simulink model "PEMFC_smlkCH4"  (R2015b)
settings: Solver=VariableStepAuto  StartTime=0.0  StopTime=tf  MinStep=1e-6  RelTol=1e-3
values from neighbouring files (symbols this model uses):
  A_cell = 238    [PEMFC_H2O2polarization.m]    (also in PEMFC_begin.m)
  B = 0.016    [PEMFC_CH4data.m]    (also in PEMFC_H2O2data.m = 0.005; PEMFC_H2O2polarization.m = 0.005; PEMFC_H2O2polfitting.m = 0.005; PEMFC_H2data.m)
  c_cw = 4.18e03    (= 4180)    [PEMFC_CH4data.m]    (also in PEMFC_H2O2data.m; PEMFC_H2data.m)
  c_O2 = p_O2 / (5.08e06 * exp(-498 / T))    [PEMFC_CH4data.m]    (also in PEMFC_H2O2data.m = pO2avg / (5.08e06 * exp(-498 / T)); PEMFC_H2O2polarization.m = pO2avg / (5.08e06 * exp(-498 / T(i))); PEMFC_H2O2polfitting.m = pO2avg / (5.08e06 * exp(-498 / T(i))); PEMFC_H2data.m)
  C_th = 350e03    (= 350000)    [PEMFC_CH4data.m]    (also in PEMFC_H2O2data.m; PEMFC_H2data.m)
  chi1 = 0.00129697    [PEMFC_CH4data.m]    (also in PEMFC_H2O2data.m; PEMFC_H2data.m)
  chi2 = - 1.529053    (= -1.529053)    [PEMFC_CH4data.m]    (also in PEMFC_H2O2data.m; PEMFC_H2data.m)
  chi3 = 681.731481    [PEMFC_CH4data.m]    (also in PEMFC_H2O2data.m; PEMFC_H2data.m)
  chi4 = - 136025.0    (= -136025)    [PEMFC_CH4data.m]    (also in PEMFC_H2O2data.m; PEMFC_H2data.m)
  chi5 = 10234070.7    [PEMFC_CH4data.m]    (also in PEMFC_H2O2data.m; PEMFC_H2data.m)
  CV = 4 * eta_ref    (= 3.92)    [PEMFC_CH4data.m]
  eta_ACDC = 0.92    [PEMFC_CH4data.m]    (also in PEMFC_H2data.m)
  eta_hx = 0.97    [PEMFC_CH4data.m]    (also in PEMFC_H2data.m = 0.92)
  F = 96485    [PEMFC_H2O2polarization.m]    (also in PEMFC_begin.m; PEMFC_cellstack.m)
  F_H2O = 0.5    [PEMFC_CH4data.m]    (also in PEMFC_H2data.m)
  h_airc = gamma_air * R * T / (gamma_air - 1) * ((1 / beta_c)^     ((gamma_air - 1) / gamma_air) - 1) / eta_c    [PEMFC_CH4data.m]    (also in PEMFC_H2data.m)
  h_airph = C_air * (T - T_amb) * M_air / eta_ph    [PEMFC_CH4data.m]    (also in PEMFC_H2data.m)
  h_CH4c = gamma_CH4 * R * T / (gamma_CH4 - 1) * ((1 / beta_c)^     ((gamma_CH4 - 1) / gamma_CH4) - 1) / eta_c    [PEMFC_CH4data.m]
  h_CH4ref = (h_CH4out - h_CH4in) / 0.97 * M_CH4    [PEMFC_CH4data.m]
  h_CO2pc = (h_CO2comb - h_CO2exh) / 1000 * M_CO2    [PEMFC_CH4data.m]
  h_CO2rec = (h_CO2rec_in - h_CO2_T) / 1000 * M_CO2 * eta_ref    [PEMFC_CH4data.m]
  h_cond = 500    [PEMFC_CH4data.m]    (also in PEMFC_H2O2data.m; PEMFC_H2data.m)
  h_conv = 0.1    [PEMFC_CH4data.m]    (also in PEMFC_H2O2data.m; PEMFC_H2data.m)
  h_H2Opc = C_H2Ocomb * (Tcomb - Texh) / 1000 * M_H2O    [PEMFC_CH4data.m]    (also in PEMFC_H2data.m)
  h_H2Opcvap = WaterEnthalpyVaporization (pcomb, T)    [PEMFC_CH4data.m]    (also in PEMFC_H2data.m)
  h_H2Orec = C_H2Orec * (T_ref - T) / 1000 * M_CO2 * eta_ref    [PEMFC_CH4data.m]
  h_H2Oref = (h_H2Oref_out - h_H2Oref_in) / 0.97 * M_H2O    [PEMFC_CH4data.m]
  h_H2rec = (h_H2rec_in - h_H2_T) / 1000 * M_CO2 * eta_ref    [PEMFC_CH4data.m]
  h_N2pc = (h_N2comb - h_N2exh) / 1000 * M_H2    [PEMFC_CH4data.m]    (also in PEMFC_H2data.m)
  h_O2pc = (h_O2comb - h_O2exh) / 1000 * M_O2    [PEMFC_CH4data.m]    (also in PEMFC_H2data.m)
  h_ref = - h_CH4ref - h_COref    (= 165000)    [PEMFC_CH4data.m]
  h_WHSG = h_H2OWH + h_H2Ovap    [PEMFC_CH4data.m]    (also in PEMFC_H2data.m)
  i_max = 1.2    [PEMFC_CH4data.m]    (also in PEMFC_H2O2data.m = 2.027; PEMFC_H2data.m; PEMFC_cellstack.m = 1.5)
  K_H2 = 0.04220    (= 0.0422)    [PEMFC_CH4data.m]    (also in PEMFC_H2O2data.m = pH2out / nH2out; PEMFC_H2data.m)
  K_O2 = 0.02110    (= 0.0211)    [PEMFC_CH4data.m]    (also in PEMFC_H2O2data.m = pO2out / nO2out; PEMFC_H2data.m)
  K_r = N_cell / (4 * F)    [PEMFC_CH4data.m]    (also in PEMFC_H2O2data.m; PEMFC_H2data.m)
  lambda = 0.90    (= 0.9)    [PEMFC_begin.m]
  m_cw = 0.25000    (= 0.25)    [PEMFC_CH4data.m]    (also in PEMFC_H2O2data.m; PEMFC_H2data.m)
  M_H2O = 18    [PEMFC_CH4data.m]    (also in PEMFC_H2O2data.m; PEMFC_H2data.m)
  N_cell = 178    [PEMFC_H2O2polarization.m]    (also in PEMFC_begin.m)
  p_cat = p_atm * 3.50    (= 3.5)    [PEMFC_H2O2polarization.m]    (also in PEMFC_begin.m)
  P_gamma = 150.0    (= 150)    [PEMFC_CH4data.m]    (also in PEMFC_H2O2data.m = 100; PEMFC_H2data.m = 155)
  p_H20 = y_H2_ref * p_an    [PEMFC_CH4data.m]    (also in PEMFC_H2O2data.m = (1 - xH2O_H2) * p_an; PEMFC_H2O2polarization.m = (1 - xH2O_H2) * p_an; PEMFC_H2O2polfitting.m = (1 - xH2O_H2) * p_an; PEMFC_H2data.m)
  p_O20 = x_O2 * p_cat    [PEMFC_CH4data.m]    (also in PEMFC_H2O2data.m = (1 - xH2O_O2) * p_cat; PEMFC_H2O2polarization.m = (1 - xH2O_O2) * p_cat; PEMFC_H2O2polfitting.m = (1 - xH2O_O2) * p_cat; PEMFC_H2data.m)
  psi = 23    [PEMFC_CH4data.m]    (also in PEMFC_H2O2data.m; PEMFC_H2O2polarization.m; PEMFC_H2O2polfitting.m; PEMFC_H2data.m)
  R_el = 0.00016    [PEMFC_CH4data.m]    (also in PEMFC_H2O2data.m = 0.00025492; PEMFC_H2data.m)
  R_th = 0.0817    [PEMFC_CH4data.m]    (also in PEMFC_H2O2data.m; PEMFC_H2data.m)
  SC = 2.50    (= 2.5)    [PEMFC_CH4data.m]
  split_CH4 = 0.30    (= 0.3)    [PEMFC_CH4data.m]
  T = [25 35 55 75 95] + 273.15    [PEMFC_H2O2polarization.m]    (also in PEMFC_begin.m = 347.15)
  T0 = T_a    [PEMFC_CH4data.m]    (also in PEMFC_H2O2data.m; PEMFC_H2data.m)
  T_a = 25    [PEMFC_begin.m]
  T_cwin = 20 + 0    (= 20)    [PEMFC_CH4data.m]    (also in PEMFC_H2O2data.m; PEMFC_H2data.m)
  T_des = T - 273.15    [PEMFC_CH4data.m]    (also in PEMFC_H2O2data.m; PEMFC_H2data.m)
  tau1_ref = 2.00    (= 2)    [PEMFC_CH4data.m]
  tau2_ref = 2.00    (= 2)    [PEMFC_CH4data.m]
  tau_c = 0.10    (= 0.1)    [PEMFC_CH4data.m]    (also in PEMFC_H2data.m)
  tau_H2 = 3.37    [PEMFC_CH4data.m]    (also in PEMFC_H2O2data.m = 0.27; PEMFC_H2data.m)
  tau_hx = 15.0    (= 15)    [PEMFC_CH4data.m]    (also in PEMFC_H2data.m)
  tau_O2 = 6.74    [PEMFC_CH4data.m]    (also in PEMFC_H2O2data.m = 0.47; PEMFC_H2data.m)
  tau_ph = 2.00    (= 2)    [PEMFC_CH4data.m]    (also in PEMFC_H2data.m = 3)
  tau_th = C_th * R_th    (= 28595)    [PEMFC_CH4data.m]    (also in PEMFC_H2O2data.m; PEMFC_H2data.m)
  tau_WHSG = 40.00    (= 40)    [PEMFC_CH4data.m]    (also in PEMFC_H2data.m = 50)
  U = polyval(polU, n_CH4in(1))    [PEMFC_CH4data.m]    (also in PEMFC_H2O2polarization.m = extractfield(V, b2)'; PEMFC_H2O2polfitting.m = extractfield(V, b2)'; PEMFC_H2data.m = polyval(polU, n_H2in(1)))
  V_tn = 1.48    [PEMFC_CH4data.m]    (also in PEMFC_H2O2data.m = 1.253; PEMFC_H2data.m)
  x_H2O = p_H2Ovap / p_cat    [PEMFC_CH4data.m]    (also in PEMFC_H2data.m)
  x_H2Ovap = WaterSaturationPressure (Texh) / pcomb    [PEMFC_CH4data.m]    (also in PEMFC_H2data.m)
  x_O2 = 0.21    [PEMFC_begin.m]
  xi1 = -0.949    [PEMFC_CH4data.m]    (also in PEMFC_H2O2data.m = -0.61693; PEMFC_H2O2polarization.m = xi(1); PEMFC_H2data.m; PEMFC_cellstack.m)
  xi2 = 0.003420    (= 0.00342)    [PEMFC_CH4data.m]    (also in PEMFC_H2O2data.m = 0.0016838; PEMFC_H2O2polarization.m = xi(2); PEMFC_H2data.m; PEMFC_cellstack.m)
  xi3 = 7.6e-05    [PEMFC_CH4data.m]    (also in PEMFC_H2O2data.m = 1.9385e-06; PEMFC_H2O2polarization.m = xi(3); PEMFC_H2data.m; PEMFC_cellstack.m)
  xi4 = -1.93e-04    (= -0.000193)    [PEMFC_CH4data.m]    (also in PEMFC_H2O2data.m = -6.4922e-05; PEMFC_H2O2polarization.m = xi(4); PEMFC_H2data.m; PEMFC_cellstack.m)
  y_CO2_ref = 1 - y_H2_ref - y_H2O_ref    [PEMFC_CH4data.m]    (also in PEMFC_H2data.m)
  y_H2_ref = 0.66    [PEMFC_begin.m]
  y_H2O_ref = 0.15    [PEMFC_begin.m]
  z_m = 178e-04    (= 0.0178)    [PEMFC_CH4data.m]    (also in PEMFC_H2O2polarization.m = 0.003; PEMFC_H2data.m; PEMFC_begin.m = 0.003; PEMFC_cellstack.m)
settings Model: Creator=gapaolo  LastModifiedBy=gapaolo

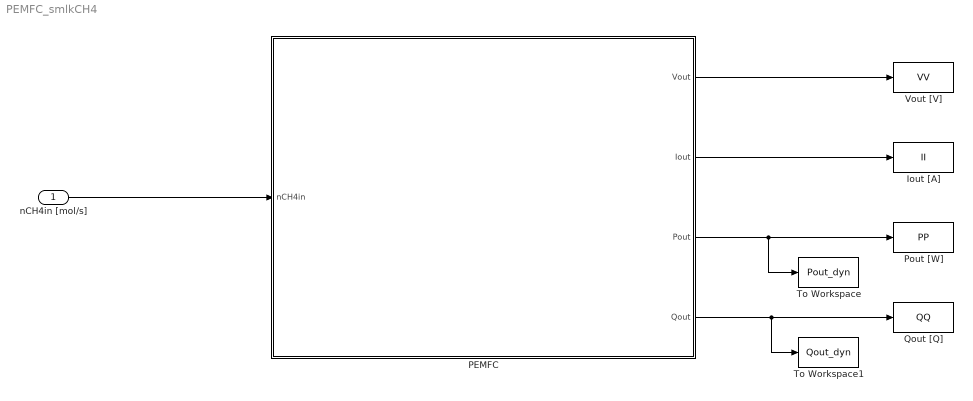
== system PEMFC_smlkCH4 ==
  nCH4in [mol/s] : Inport
  Iout [A] : ToWorkspace  VariableName=II  SaveFormat=Timeseries  SampleTime=-1
  PEMFC : Subsystem
  Pout [W] : ToWorkspace  VariableName=PP  SaveFormat=Timeseries  SampleTime=-1
  Qout [Q] : ToWorkspace  VariableName=QQ  SaveFormat=Timeseries  SampleTime=-1
  To Workspace : ToWorkspace  VariableName=Pout_dyn  SaveFormat=Timeseries  SampleTime=-1
  To Workspace1 : ToWorkspace  VariableName=Qout_dyn  SaveFormat=Timeseries  SampleTime=-1
  Vout [V] : ToWorkspace  VariableName=VV  SaveFormat=Timeseries  SampleTime=-1
  wires:
  nCH4in [mol/s]/1 -> PEMFC/1(nCH4in)
  PEMFC/1(Vout) -> Vout [V]/1
  PEMFC/2(Iout) -> Iout [A]/1
  PEMFC/4(Qout) -> To Workspace1/1, Qout [Q]/1
  PEMFC/3(Pout) -> To Workspace/1, Pout [W]/1

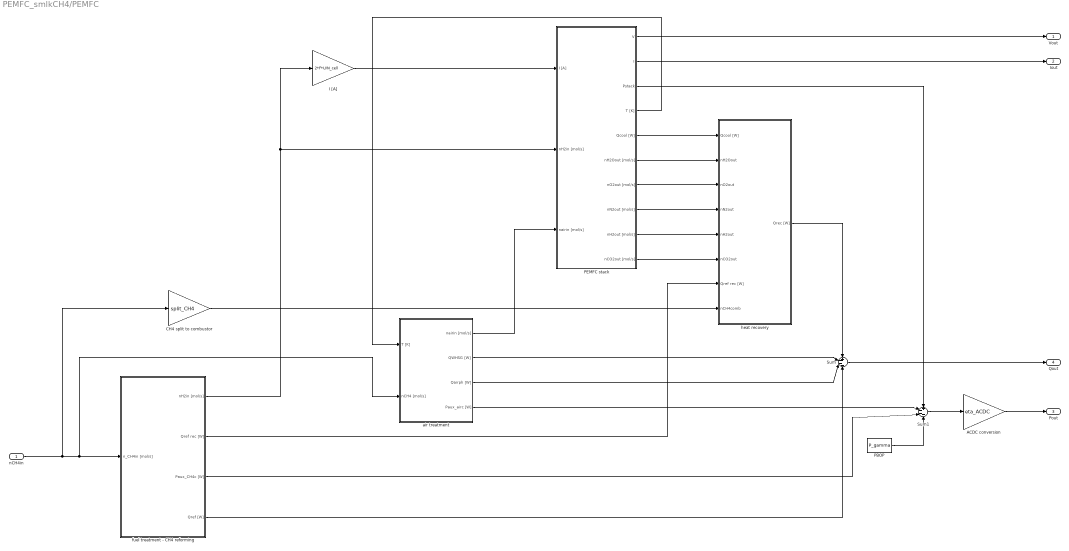
== system PEMFC_smlkCH4/PEMFC ==
  nCH4in : Inport
  ACDC conversion : Gain  Gain=eta_ACDC
  CH4 split to combustor : Gain  Gain=split_CH4
  I [A] : Gain  Gain=2*F*U/N_cell
  PBOP : Constant  Value=P_gamma
  PEMFC stack : Subsystem
  Sum : Sum  Inputs=+---
  Sum1 : Sum  Inputs=+---
  air treatment : Subsystem
  fuel treatment - CH4 reforming : Subsystem
  heat recovery : Subsystem
  Vout : Outport
  Iout : Outport  Port=2
  Pout : Outport  Port=3
  Qout : Outport  Port=4
  wires:
  fuel treatment - CH4 reforming/1(nH2in [mol/s]) -> I [A]/1, PEMFC stack/2(nH2in [mol/s])
  I [A]/1 -> PEMFC stack/1(I [A])
  air treatment/1(nairin [mol/s]) -> PEMFC stack/3(nairin [mol/s])
  PEMFC stack/1("V ") -> Vout/1
  PEMFC stack/2(I) -> Iout/1
  PEMFC stack/4(T [K]) -> air treatment/1(T [K])
  PEMFC stack/3(Pstack) -> Sum1/1
  PEMFC stack/5(Qcool [W]) -> heat recovery/1(Qcool [W])
  fuel treatment - CH4 reforming/2(Qref rec [W]) -> heat recovery/7(Qref rec [W])
  PEMFC stack/6(nH2Oout [mol/s]) -> heat recovery/2(nH2Oout)
  PEMFC stack/7(nO2out [mol/s]) -> heat recovery/3(nO2out)
  PEMFC stack/8(nN2out [mol/s]) -> heat recovery/4(nN2out)
  PEMFC stack/9(nH2out [mol/s]) -> heat recovery/5(nH2out)
  PEMFC stack/10(nCO2out [mol/s]) -> heat recovery/6(nCO2out)
  CH4 split to combustor/1 -> heat recovery/8(nCH4comb)
  Sum1/1 -> ACDC conversion/1
  heat recovery/1(Qrec [W]) -> Sum/1
  fuel treatment - CH4 reforming/3(Paux_CH4c [W]) -> Sum1/3
  air treatment/3(Qairph [W]) -> Sum/3
  air treatment/4(Paux_airc [W]) -> Sum1/2
  air treatment/2(QWHSG [W]) -> Sum/2
  fuel treatment - CH4 reforming/4(Qref [W]) -> Sum/4
  nCH4in/1 -> CH4 split to combustor/1, air treatment/2(nCH4 [mol/s]), fuel treatment - CH4 reforming/1(n_CH4in [mol/s])
  PBOP/1 -> Sum1/4
  ACDC conversion/1 -> Pout/1
  Sum/1 -> Qout/1

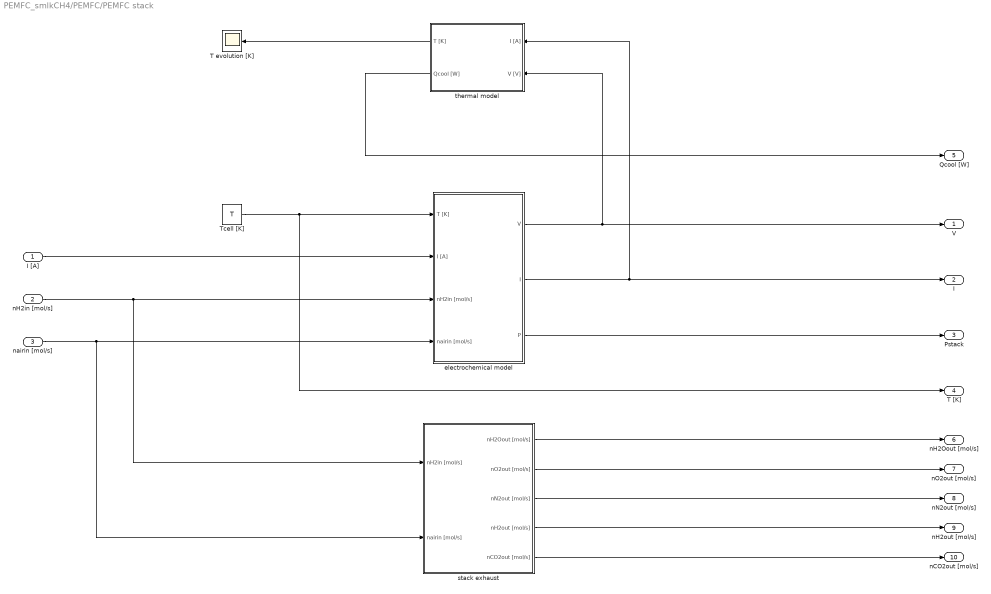
== system PEMFC_smlkCH4/PEMFC/PEMFC stack ==
  I [A] : Inport
  nH2in [mol/s] : Inport  Port=2
  nairin [mol/s] : Inport  Port=3
  T evolution [K] : Scope
  Tcell [K] : Constant  Value=T
  electrochemical model : Subsystem
  stack exhaust : Subsystem
  thermal model : Subsystem
  "V " : Outport
  I : Outport  Port=2
  Pstack : Outport  Port=3
  T [K] : Outport  Port=4
  Qcool [W] : Outport  Port=5
  nH2Oout [mol/s] : Outport  Port=6
  nO2out [mol/s] : Outport  Port=7
  nN2out [mol/s] : Outport  Port=8
  nH2out [mol/s] : Outport  Port=9
  nCO2out [mol/s] : Outport  Port=10
  wires:
  nairin [mol/s]/1 -> stack exhaust/2(nairin [mol/s]), electrochemical model/4(nairin [mol/s])
  electrochemical model/3(P) -> Pstack/1
  nH2in [mol/s]/1 -> electrochemical model/3(nH2in [mol/s]), stack exhaust/1(nH2in [mol/s])
  stack exhaust/1(nH2Oout [mol/s]) -> nH2Oout [mol/s]/1
  stack exhaust/2(nO2out [mol/s]) -> nO2out [mol/s]/1
  stack exhaust/3(nN2out [mol/s]) -> nN2out [mol/s]/1
  stack exhaust/4(nH2out [mol/s]) -> nH2out [mol/s]/1
  stack exhaust/5(nCO2out [mol/s]) -> nCO2out [mol/s]/1
  Tcell [K]/1 -> T [K]/1, electrochemical model/1(T [K])
  thermal model/1(T [K]) -> T evolution [K]/1
  I [A]/1 -> electrochemical model/2("I [A] ")
  thermal model/2(Qcool [W]) -> Qcool [W]/1
  electrochemical model/2(I) -> I/1, thermal model/1(I [A])
  electrochemical model/1(V) -> thermal model/2(V [V]), "V "/1

== system PEMFC_smlkCH4/PEMFC/air treatment ==
  T [K] : Inport
  nCH4 [mol/s] : Inport  Port=2
  CH4 --> H2 : Gain  Gain=CV
  Sum1 : Sum  Inputs=++|
  Water vaporization : Subsystem
  air humdifier : Subsystem
  auxiliaries - air compressor and preheater : Subsystem
  nairin [mol/s] : Outport
  QWHSG [W] : Outport  Port=2
  Qairph [W] : Outport  Port=3
  Paux_airc [W] : Outport  Port=4
  wires:
  nCH4 [mol/s]/1 -> CH4 --> H2/1
  T [K]/1 -> air humdifier/2(T [K])
  air humdifier/2(nair dry [mol/s]) -> auxiliaries - air compressor and preheater/1(nair dry [mol/s])
  auxiliaries - air compressor and preheater/2(Qairph [W]) -> Qairph [W]/1
  auxiliaries - air compressor and preheater/3(Paux_airc [W]) -> Paux_airc [W]/1
  auxiliaries - air compressor and preheater/1(nair dry) -> Sum1/2
  Sum1/1 -> nairin [mol/s]/1
  air humdifier/1(nH2O [mol/s]) -> Water vaporization/1(nH2O [mol/s])
  Water vaporization/1(QWHSG) -> QWHSG [W]/1
  Water vaporization/2(nH2O) -> Sum1/1
  CH4 --> H2/1 -> air humdifier/1(nH2 [mol/s])

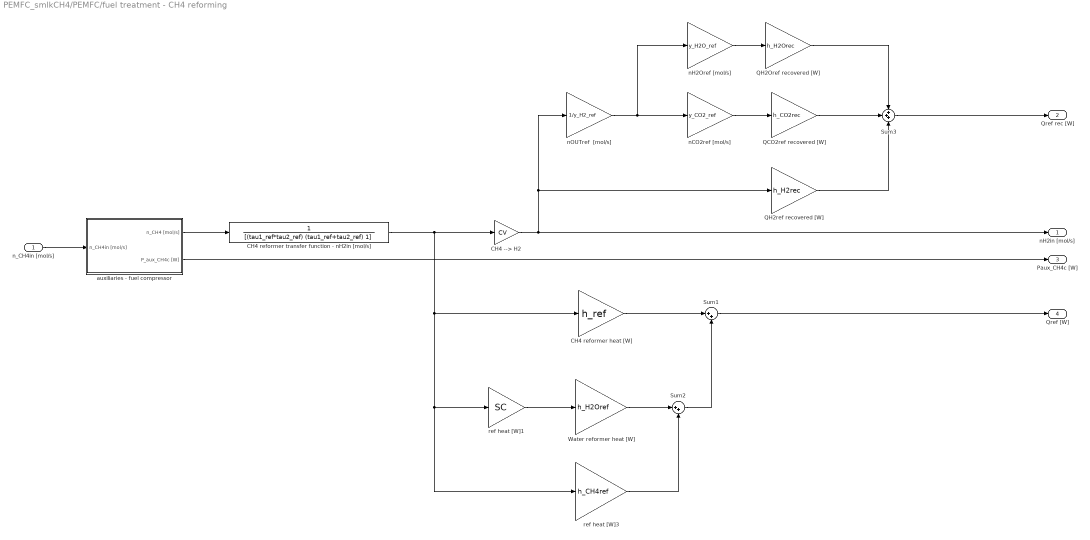
== system PEMFC_smlkCH4/PEMFC/fuel treatment - CH4 reforming ==
  n_CH4in [mol/s] : Inport
  CH4 --> H2 : Gain  Gain=CV
  CH4 reformer heat [W] : Gain  Gain=h_ref
  CH4 reformer transfer function - nH2in [mol/s] : TransferFcn  Denominator=[(tau1_ref*tau2_ref) (tau1_ref+tau2_ref) 1]  ContinuousStateAttributes='q_H2'
  QCO2ref recovered [W] : Gain  Gain=h_CO2rec
  QH2Oref recovered [W] : Gain  Gain=h_H2Orec
  QH2ref recovered [W] : Gain  Gain=h_H2rec
  Sum1 : Sum  Inputs=|++
  Sum2 : Sum  Inputs=|++
  Sum3 : Sum  Inputs=+++
  Water reformer heat [W] : Gain  Gain=h_H2Oref
  auxiliaries - fuel compressor : Subsystem
  nCO2ref [mol/s] : Gain  Gain=y_CO2_ref
  nH2Oref [mol/s] : Gain  Gain=y_H2O_ref
  "nOUTref  [mol/s] " : Gain  Gain=1/y_H2_ref
  ref heat [W]1 : Gain  Gain=SC
  ref heat [W]3 : Gain  Gain=h_CH4ref
  nH2in [mol/s] : Outport
  Qref rec [W] : Outport  Port=2
  Paux_CH4c [W] : Outport  Port=3
  Qref [W] : Outport  Port=4
  wires:
  CH4 reformer transfer function - nH2in [mol/s]/1 -> ref heat [W]3/1, ref heat [W]1/1, CH4 reformer heat [W]/1, CH4 --> H2/1
  auxiliaries - fuel compressor/2(P_aux_CH4c [W]) -> Paux_CH4c [W]/1
  CH4 --> H2/1 -> "nOUTref  [mol/s] "/1, QH2ref recovered [W]/1, nH2in [mol/s]/1
  auxiliaries - fuel compressor/1(n_CH4 [mol/s]) -> CH4 reformer transfer function - nH2in [mol/s]/1
  Sum2/1 -> Sum1/2
  ref heat [W]3/1 -> Sum2/2
  ref heat [W]1/1 -> Water reformer heat [W]/1
  CH4 reformer heat [W]/1 -> Sum1/1
  Water reformer heat [W]/1 -> Sum2/1
  Sum1/1 -> Qref [W]/1
  n_CH4in [mol/s]/1 -> auxiliaries - fuel compressor/1(n_CH4in [mol/s])
  "nOUTref  [mol/s] "/1 -> nH2Oref [mol/s]/1, nCO2ref [mol/s]/1
  nH2Oref [mol/s]/1 -> QH2Oref recovered [W]/1
  nCO2ref [mol/s]/1 -> QCO2ref recovered [W]/1
  QCO2ref recovered [W]/1 -> Sum3/2
  QH2Oref recovered [W]/1 -> Sum3/1
  QH2ref recovered [W]/1 -> Sum3/3
  Sum3/1 -> Qref rec [W]/1

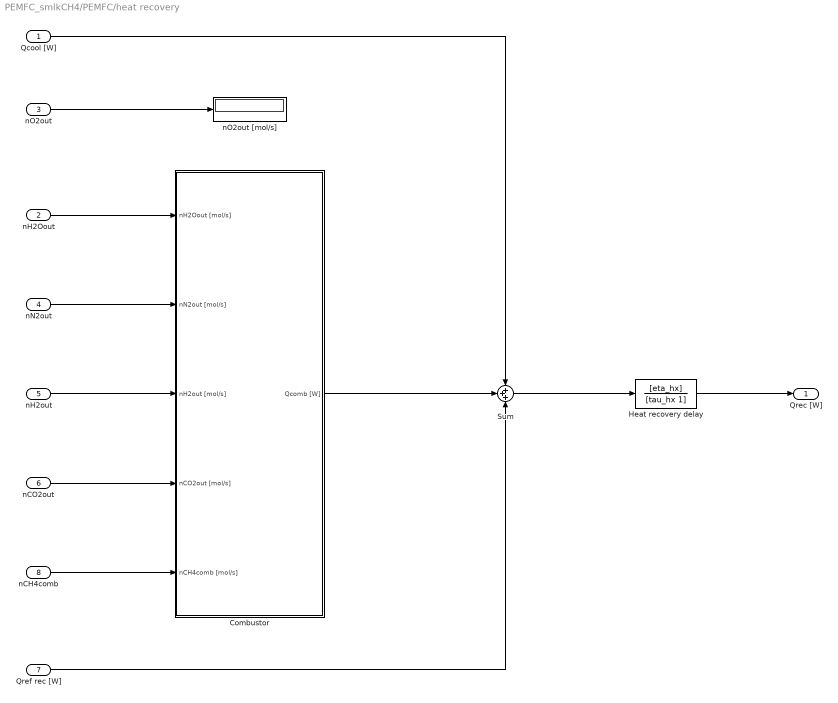
== system PEMFC_smlkCH4/PEMFC/heat recovery ==
  Qcool [W] : Inport
  nH2Oout : Inport  Port=2
  nO2out : Inport  Port=3
  nN2out : Inport  Port=4
  nH2out : Inport  Port=5
  nCO2out : Inport  Port=6
  Qref rec [W] : Inport  Port=7
  nCH4comb : Inport  Port=8
  Combustor : Subsystem
  Heat recovery delay : TransferFcn  Numerator=[eta_hx]  Denominator=[tau_hx 1]
  Sum : Sum  Inputs=+++
  nO2out [mol/s] : Display
  Qrec [W] : Outport
  wires:
  nO2out/1 -> nO2out [mol/s]/1
  nH2Oout/1 -> Combustor/1(nH2Oout [mol/s])
  nN2out/1 -> Combustor/2(nN2out [mol/s])
  nH2out/1 -> Combustor/3(nH2out [mol/s])
  nCO2out/1 -> Combustor/4(nCO2out [mol/s])
  nCH4comb/1 -> Combustor/5(nCH4comb [mol/s])
  Combustor/1(Qcomb [W]) -> Sum/2
  Qref rec [W]/1 -> Sum/3
  Qcool [W]/1 -> Sum/1
  Sum/1 -> Heat recovery delay/1
  Heat recovery delay/1 -> Qrec [W]/1

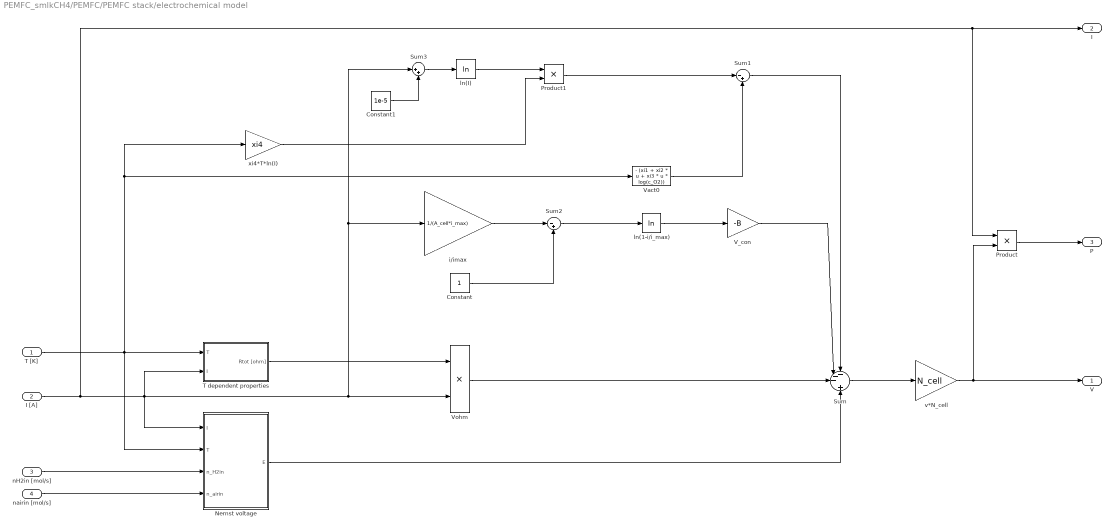
== system PEMFC_smlkCH4/PEMFC/PEMFC stack/electrochemical model ==
  T [K] : Inport
  "I [A] " : Inport  Port=2
  nH2in [mol/s] : Inport  Port=3
  nairin [mol/s] : Inport  Port=4
  Constant : Constant
  Constant1 : Constant  Value=1e-5
  Nernst voltage : Subsystem
  Product : Product
  Product1 : Product
  Sum : Sum  Inputs=---|+
  Sum1 : Sum  Inputs=|-+
  Sum2 : Sum  Inputs=|-+
  Sum3 : Sum  Inputs=|++
  T dependent properties : Subsystem
  V_con : Gain  Gain=-B
  Vact0 : Fcn  Expr=- (xi1 + xi2 * u + xi3 * u * log(c_O2))
  Vohm : Product
  i/imax : Gain  Gain=1/(A_cell*i_max)
  ln(1-i/i_max) : Math  Operator=log  SaturateOnIntegerOverflow=on
  "ln(I) " : Math  Operator=log  SaturateOnIntegerOverflow=on
  v*N_cell : Gain  Gain=N_cell
  xi4*T*ln(I) : Gain  Gain=xi4
  V : Outport
  I : Outport  Port=2
  P : Outport  Port=3
  wires:
  Sum/1 -> v*N_cell/1
  T [K]/1 -> xi4*T*ln(I)/1, Vact0/1, Nernst voltage/2(T), T dependent properties/1(T)
  T dependent properties/1(Rtot [ohm]) -> Vohm/1
  Vohm/1 -> Sum/3
  i/imax/1 -> Sum2/1
  Constant/1 -> Sum2/2
  Sum2/1 -> ln(1-i/i_max)/1
  ln(1-i/i_max)/1 -> V_con/1
  Sum1/1 -> Sum/1
  v*N_cell/1 -> Product/2, V/1
  V_con/1 -> Sum/2
  "ln(I) "/1 -> Product1/1
  Product1/1 -> Sum1/1
  Vact0/1 -> Sum1/2
  "I [A] "/1 -> Product/1, I/1, Nernst voltage/1(I), T dependent properties/2(I), Vohm/2, i/imax/1, Sum3/1
  Nernst voltage/1(E) -> Sum/4
  nH2in [mol/s]/1 -> Nernst voltage/3(n_H2in)
  nairin [mol/s]/1 -> Nernst voltage/4(n_airin)
  Product/1 -> P/1
  Sum3/1 -> "ln(I) "/1
  Constant1/1 -> Sum3/2
  xi4*T*ln(I)/1 -> Product1/2

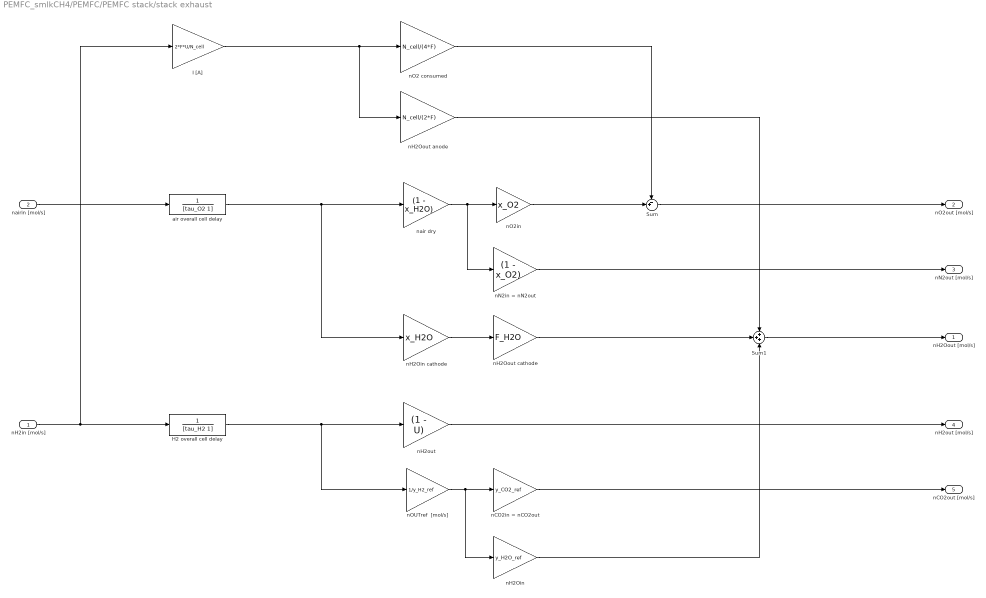
== system PEMFC_smlkCH4/PEMFC/PEMFC stack/stack exhaust ==
  nH2in [mol/s] : Inport
  nairin [mol/s] : Inport  Port=2
  H2 overall cell delay : TransferFcn  Denominator=[tau_H2 1]  ContinuousStateAttributes='p_O2'
  I [A] : Gain  Gain=2*F*U/N_cell
  Sum : Sum  Inputs=-+|
  Sum1 : Sum  Inputs=+++
  air overall cell delay : TransferFcn  Denominator=[tau_O2 1]  ContinuousStateAttributes='p_O2'
  nCO2in = nCO2out : Gain  Gain=y_CO2_ref
  nH2Oin : Gain  Gain=y_H2O_ref
  nH2Oin cathode : Gain  Gain=x_H2O
  nH2Oout anode : Gain  Gain=N_cell/(2*F)
  nH2Oout cathode : Gain  Gain=F_H2O
  nH2out : Gain  Gain=(1 - U)
  nN2in = nN2out : Gain  Gain=(1 - x_O2)
  nO2 consumed : Gain  Gain=N_cell/(4*F)
  nO2in : Gain  Gain=x_O2
  "nOUTref  [mol/s] " : Gain  Gain=1/y_H2_ref
  nair dry : Gain  Gain=(1 - x_H2O)
  nH2Oout [mol/s] : Outport
  nO2out [mol/s] : Outport  Port=2
  nN2out [mol/s] : Outport  Port=3
  nH2out [mol/s] : Outport  Port=4
  nCO2out [mol/s] : Outport  Port=5
  wires:
  nH2Oin cathode/1 -> nH2Oout cathode/1
  nair dry/1 -> nN2in = nN2out/1, nO2in/1
  nairin [mol/s]/1 -> air overall cell delay/1
  nH2in [mol/s]/1 -> I [A]/1, H2 overall cell delay/1
  nO2in/1 -> Sum/2
  nO2 consumed/1 -> Sum/1
  "nOUTref  [mol/s] "/1 -> nH2Oin/1, nCO2in = nCO2out/1
  Sum/1 -> nO2out [mol/s]/1
  nH2Oout cathode/1 -> Sum1/2
  nH2Oout anode/1 -> Sum1/1
  nH2Oin/1 -> Sum1/3
  Sum1/1 -> nH2Oout [mol/s]/1
  nN2in = nN2out/1 -> nN2out [mol/s]/1
  nH2out/1 -> nH2out [mol/s]/1
  nCO2in = nCO2out/1 -> nCO2out [mol/s]/1
  H2 overall cell delay/1 -> "nOUTref  [mol/s] "/1, nH2out/1
  air overall cell delay/1 -> nH2Oin cathode/1, nair dry/1
  I [A]/1 -> nH2Oout anode/1, nO2 consumed/1

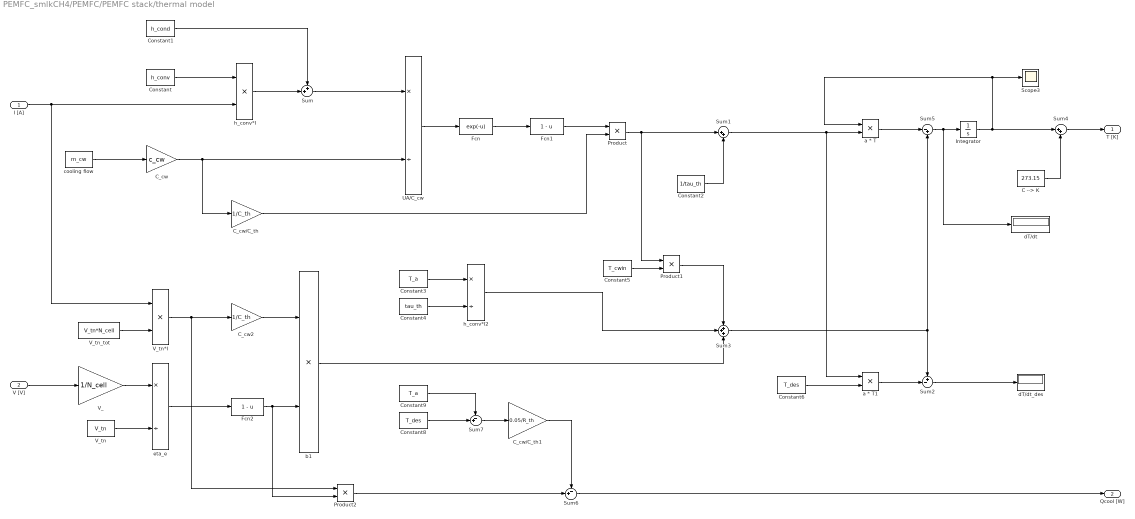
== system PEMFC_smlkCH4/PEMFC/PEMFC stack/thermal model ==
  I [A] : Inport
  V [V] : Inport  Port=2
  C --> K : Constant  Value=273.15
  C_cw : Gain  Gain=c_cw
  C_cw/C_th : Gain  Gain=1/C_th
  C_cw/C_th1 : Gain  Gain=0.05/R_th
  C_cw2 : Gain  Gain=1/C_th
  Constant : Constant  Value=h_conv
  Constant1 : Constant  Value=h_cond
  Constant2 : Constant  Value=1/tau_th
  Constant3 : Constant  Value=T_a
  Constant4 : Constant  Value=tau_th
  Constant5 : Constant  Value=T_cwin
  Constant6 : Constant  Value=T_des
  Constant8 : Constant  Value=T_des
  Constant9 : Constant  Value=T_a
  Fcn : Fcn  Expr=exp(-u)
  Fcn1 : Fcn  Expr=1 - u
  Fcn2 : Fcn  Expr=1 - u
  Integrator : Integrator  InitialCondition=T0  AbsoluteTolerance=1e-6
  Product : Product
  Product1 : Product
  Product2 : Product
  Scope3 : Scope
  Sum : Sum  Inputs=++|
  Sum1 : Sum  Inputs=|++
  Sum2 : Sum  Inputs=+-|
  Sum3 : Sum  Inputs=+++
  Sum4 : Sum  Inputs=|++
  Sum5 : Sum  Inputs=|-+
  Sum6 : Sum  Inputs=-+|
  Sum7 : Sum  Inputs=-+|
  UA/C_cw : Product  Inputs=*/
  V_ : Gain  Gain=1/N_cell
  V_tn : Constant  Value=V_tn
  V_tn*I : Product
  V_tn_tot : Constant  Value=V_tn*N_cell
  a * T : Product
  a * T1 : Product
  b1 : Product
  cooling flow : Constant  Value=m_cw
  dT/dt : Display
  dT/dt_des : Display
  eta_e : Product  Inputs=*/
  h_conv*I : Product
  h_conv*I2 : Product  Inputs=*/
  T [K] : Outport
  Qcool [W] : Outport  Port=2
  wires:
  V_tn_tot/1 -> V_tn*I/2
  eta_e/1 -> Fcn2/1
  V_tn/1 -> eta_e/2
  V_/1 -> eta_e/1
  b1/1 -> Sum3/3
  h_conv*I2/1 -> Sum3/2
  Product1/1 -> Sum3/1
  Constant5/1 -> Product1/2
  Constant4/1 -> h_conv*I2/2
  Constant3/1 -> h_conv*I2/1
  C_cw2/1 -> b1/1
  V [V]/1 -> V_/1
  Constant2/1 -> Sum1/2
  Product/1 -> Sum1/1, Product1/1
  C_cw/C_th/1 -> Product/2
  Fcn1/1 -> Product/1
  C_cw/1 -> C_cw/C_th/1, UA/C_cw/2
  Fcn/1 -> Fcn1/1
  UA/C_cw/1 -> Fcn/1
  cooling flow/1 -> C_cw/1
  Sum/1 -> UA/C_cw/1
  Constant1/1 -> Sum/1
  h_conv*I/1 -> Sum/2
  Constant/1 -> h_conv*I/1
  I [A]/1 -> h_conv*I/2, V_tn*I/1
  Integrator/1 -> Sum4/1, a * T/1, Scope3/1
  a * T/1 -> Sum5/1
  Sum3/1 -> Sum5/2, Sum2/1
  Sum1/1 -> a * T1/1, a * T/2
  Constant6/1 -> a * T1/2
  a * T1/1 -> Sum2/2
  Sum2/1 -> dT/dt_des/1
  C --> K/1 -> Sum4/2
  Sum4/1 -> T [K]/1
  Product2/1 -> Sum6/2
  Constant8/1 -> Sum7/2
  Constant9/1 -> Sum7/1
  Sum7/1 -> C_cw/C_th1/1
  C_cw/C_th1/1 -> Sum6/1
  Sum6/1 -> Qcool [W]/1
  V_tn*I/1 -> Product2/1, C_cw2/1
  Fcn2/1 -> Product2/2, b1/2
  Sum5/1 -> dT/dt/1, Integrator/1

== system PEMFC_smlkCH4/PEMFC/air treatment/Water vaporization ==
  nH2O [mol/s] : Inport
  Q_WHSG [W] : Gain  Gain=h_WHSG
  WHSG delay : TransferFcn  Denominator=[tau_WHSG 1]
  mH2O [g/s] : Gain  Gain=M_H2O
  nH2Odelay [mol/s] : Gain  Gain=1/h_WHSG/M_H2O
  QWHSG : Outport
  nH2O : Outport  Port=2
  wires:
  mH2O [g/s]/1 -> Q_WHSG [W]/1
  Q_WHSG [W]/1 -> WHSG delay/1
  nH2O [mol/s]/1 -> mH2O [g/s]/1
  WHSG delay/1 -> QWHSG/1, nH2Odelay [mol/s]/1
  nH2Odelay [mol/s]/1 -> nH2O/1

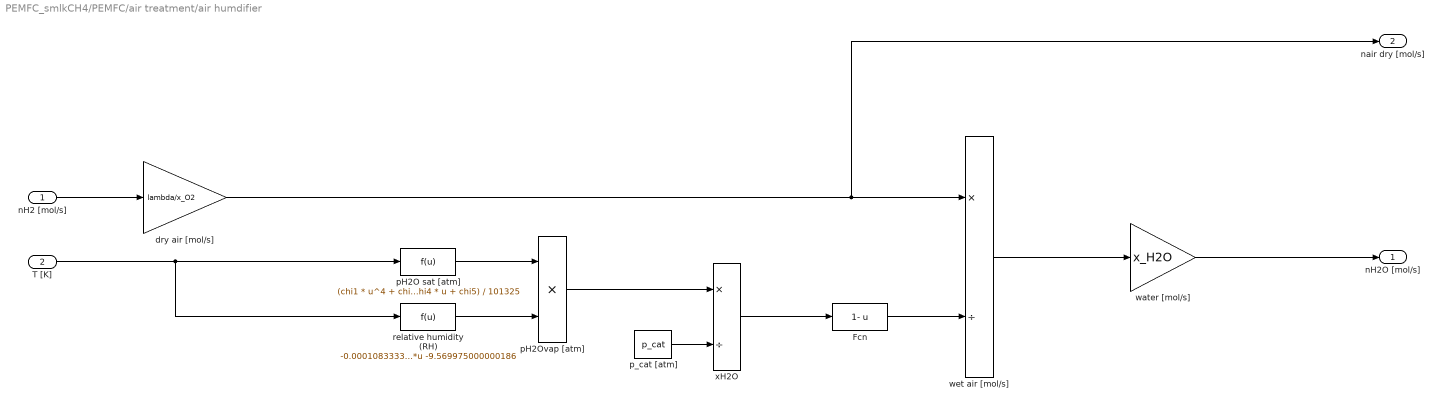
== system PEMFC_smlkCH4/PEMFC/air treatment/air humdifier ==
  nH2 [mol/s] : Inport
  T [K] : Inport  Port=2
  Fcn : Fcn  Expr=1- u
  dry air [mol/s] : Gain  Gain=lambda/x_O2
  pH2O sat [atm] : Fcn  Expr=(chi1 * u^4 + chi2 * u^3 + chi3 * u^2 + chi4 * u + chi5) / 101325
  pH2Ovap [atm] : Product
  p_cat [atm] : Constant  Value=p_cat
  relative humidity (RH) : Fcn  Expr=-0.000108333333333*u^2 + 0.067816666666668*u -9.569975000000186
  water [mol/s] : Gain  Gain=x_H2O
  wet air [mol/s] : Product  Inputs=*/
  xH2O : Product  Inputs=*/
  nH2O [mol/s] : Outport
  nair dry [mol/s] : Outport  Port=2
  wires:
  Fcn/1 -> wet air [mol/s]/2
  xH2O/1 -> Fcn/1
  dry air [mol/s]/1 -> nair dry [mol/s]/1, wet air [mol/s]/1
  wet air [mol/s]/1 -> water [mol/s]/1
  nH2 [mol/s]/1 -> dry air [mol/s]/1
  pH2Ovap [atm]/1 -> xH2O/1
  pH2O sat [atm]/1 -> pH2Ovap [atm]/1
  relative humidity (RH)/1 -> pH2Ovap [atm]/2
  p_cat [atm]/1 -> xH2O/2
  T [K]/1 -> relative humidity (RH)/1, pH2O sat [atm]/1
  water [mol/s]/1 -> nH2O [mol/s]/1

== system PEMFC_smlkCH4/PEMFC/air treatment/auxiliaries - air compressor and preheater ==
  nair dry [mol/s] : Inport
  Paux_airc : Gain  Gain=h_airc
  Qairph : Gain  Gain=h_airph
  air preheating delay : TransferFcn  Denominator=[tau_ph 1]
  nair dry delay : Gain  Gain=1/h_airph
  nair dry : Outport
  Qairph [W] : Outport  Port=2
  Paux_airc [W] : Outport  Port=3
  wires:
  nair dry [mol/s]/1 -> Qairph/1, Paux_airc/1
  Paux_airc/1 -> Paux_airc [W]/1
  Qairph/1 -> air preheating delay/1
  nair dry delay/1 -> nair dry/1
  air preheating delay/1 -> Qairph [W]/1, nair dry delay/1

== system PEMFC_smlkCH4/PEMFC/fuel treatment - CH4 reforming/auxiliaries - fuel compressor ==
  n_CH4in [mol/s] : Inport
  CH4 compression delay : TransferFcn  Denominator=[tau_c 1]
  CH4 compression work : Gain  Gain=h_CH4c
  CH4 mole flow : Gain  Gain=1/h_CH4c
  n_CH4 [mol/s] : Outport
  P_aux_CH4c [W] : Outport  Port=2
  wires:
  CH4 compression work/1 -> CH4 compression delay/1
  n_CH4in [mol/s]/1 -> CH4 compression work/1
  CH4 mole flow/1 -> n_CH4 [mol/s]/1
  CH4 compression delay/1 -> CH4 mole flow/1, P_aux_CH4c [W]/1

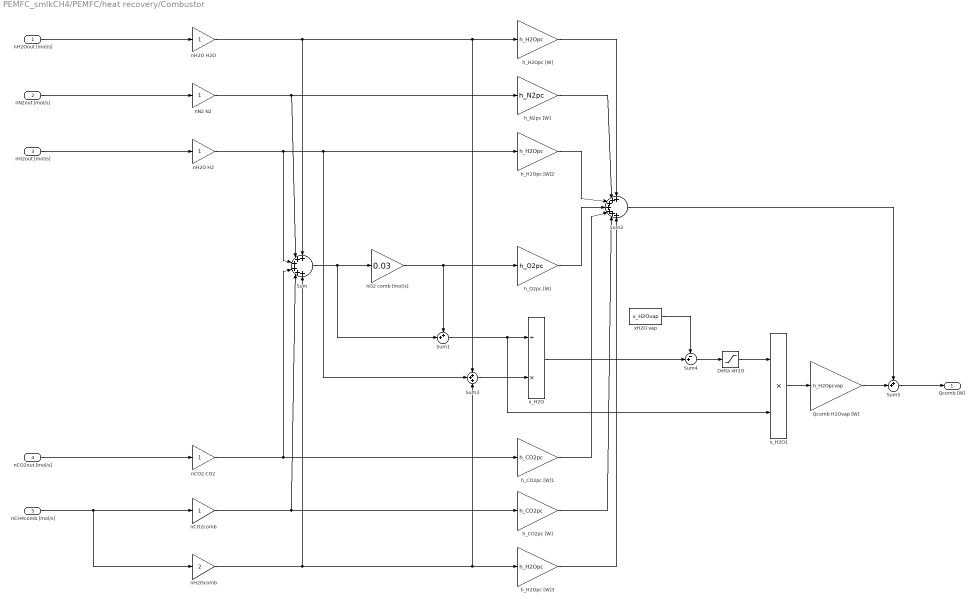
== system PEMFC_smlkCH4/PEMFC/heat recovery/Combustor ==
  nH2Oout [mol/s] : Inport
  nN2out [mol/s] : Inport  Port=2
  nH2out [mol/s] : Inport  Port=3
  nCO2out [mol/s] : Inport  Port=4
  nCH4comb [mol/s] : Inport  Port=5
  Delta xH2O : Saturate  UpperLimit=1  LowerLimit=0
  Qcomb H2Ovap [W] : Gain  Gain=h_H2Opcvap
  Sum : Sum  Inputs=++++++
  Sum1 : Sum  Inputs=++|
  Sum2 : Sum  Inputs=+++++++
  Sum3 : Sum  Inputs=+++
  Sum4 : Sum  Inputs=-+|
  Sum5 : Sum  Inputs=++|
  h_CO2pc [W] : Gain  Gain=h_CO2pc
  h_CO2pc [W]1 : Gain  Gain=h_CO2pc
  h_H2Opc [W] : Gain  Gain=h_H2Opc
  h_H2Opc [W]2 : Gain  Gain=h_H2Opc
  h_H2Opc [W]3 : Gain  Gain=h_H2Opc
  h_N2pc [W] : Gain  Gain=h_N2pc
  h_O2pc [W] : Gain  Gain=h_O2pc
  nCO2 CO2 : Gain
  nCO2comb : Gain
  nH2O H2 : Gain
  nH2O H2O : Gain
  nH2Ocomb : Gain  Gain=2
  nN2 N2 : Gain
  nO2 comb [mol/s] : Gain  Gain=0.03
  xH2O vap : Constant  Value=x_H2Ovap
  x_H2O : Product  Inputs=/*
  x_H2O1 : Product  Inputs=**
  Qcomb [W] : Outport
  wires:
  h_H2Opc [W]/1 -> Sum2/1
  Sum2/1 -> Sum5/1
  h_CO2pc [W]/1 -> Sum2/6
  h_H2Opc [W]3/1 -> Sum2/7
  h_H2Opc [W]2/1 -> Sum2/3
  Sum5/1 -> Qcomb [W]/1
  h_O2pc [W]/1 -> Sum2/4
  h_N2pc [W]/1 -> Sum2/2
  nO2 comb [mol/s]/1 -> Sum1/1, h_O2pc [W]/1
  nCH4comb [mol/s]/1 -> nH2Ocomb/1, nCO2comb/1
  nCO2out [mol/s]/1 -> nCO2 CO2/1
  nH2out [mol/s]/1 -> nH2O H2/1
  nN2out [mol/s]/1 -> nN2 N2/1
  nH2Oout [mol/s]/1 -> nH2O H2O/1
  nCO2comb/1 -> h_CO2pc [W]/1, Sum/5
  nH2Ocomb/1 -> Sum/6, Sum3/3, h_H2Opc [W]3/1
  Sum/1 -> Sum1/2, nO2 comb [mol/s]/1
  nH2O H2O/1 -> Sum/1, Sum3/1, h_H2Opc [W]/1
  nN2 N2/1 -> h_N2pc [W]/1, Sum/2
  nH2O H2/1 -> Sum3/2, h_H2Opc [W]2/1, Sum/3
  nCO2 CO2/1 -> h_CO2pc [W]1/1, Sum/4
  Sum3/1 -> x_H2O/2
  Sum1/1 -> x_H2O1/2, x_H2O/1
  xH2O vap/1 -> Sum4/1
  Sum4/1 -> Delta xH2O/1
  Qcomb H2Ovap [W]/1 -> Sum5/2
  x_H2O/1 -> Sum4/2
  Delta xH2O/1 -> x_H2O1/1
  x_H2O1/1 -> Qcomb H2Ovap [W]/1
  h_CO2pc [W]1/1 -> Sum2/5

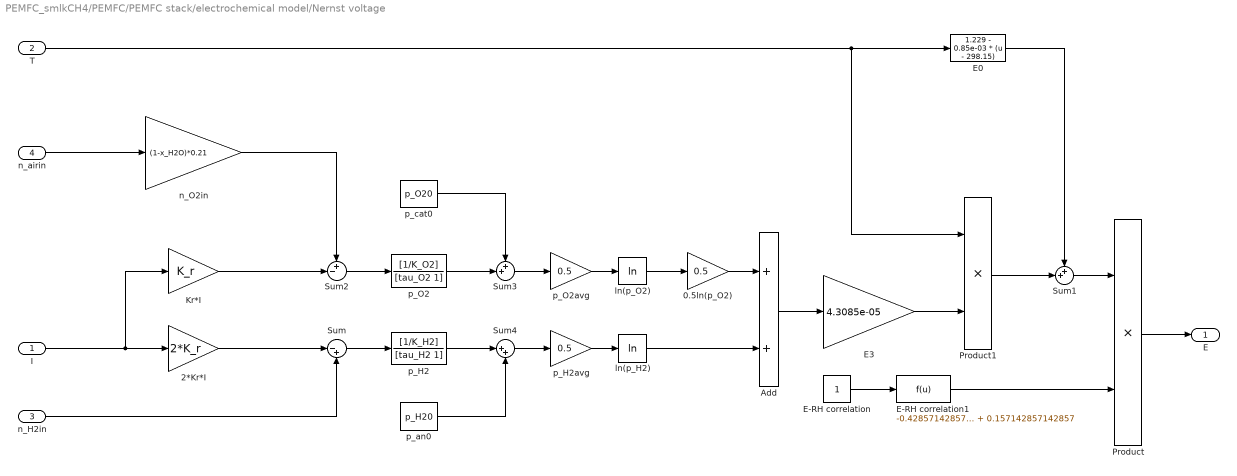
== system PEMFC_smlkCH4/PEMFC/PEMFC stack/electrochemical model/Nernst voltage ==
  I : Inport
  T : Inport  Port=2
  n_H2in : Inport  Port=3
  n_airin : Inport  Port=4
  0.5ln(p_O2) : Gain  Gain=0.5
  2*Kr*I : Gain  Gain=2*K_r
  Add : Sum
  E-RH correlation : Constant
  E-RH correlation1 : Fcn  Expr=-0.428571428571430*u^2 + 1.271428571428573 * u + 0.157142857142857
  E0 : Fcn  Expr=1.229 - 0.85e-03 * (u - 298.15)
  E3 : Gain  Gain=4.3085e-05
  Kr*I : Gain  Gain=K_r
  Product : Product
  Product1 : Product
  Sum : Sum  Inputs=|-+
  Sum1 : Sum  Inputs=++|
  Sum2 : Sum  Inputs=+-|
  Sum3 : Sum  Inputs=++|
  Sum4 : Sum  Inputs=|++
  ln(p_H2) : Math  Operator=log  SaturateOnIntegerOverflow=on
  ln(p_O2) : Math  Operator=log  SaturateOnIntegerOverflow=on
  n_O2in : Gain  Gain=(1-x_H2O)*0.21
  p_H2 : TransferFcn  Numerator=[1/K_H2]  Denominator=[tau_H2 1]  ContinuousStateAttributes='p_H2'
  p_H2avg : Gain  Gain=0.5
  p_O2 : TransferFcn  Numerator=[1/K_O2]  Denominator=[tau_O2 1]  ContinuousStateAttributes='p_O2'
  p_O2avg : Gain  Gain=0.5
  p_an0 : Constant  Value=p_H20
  p_cat0 : Constant  Value=p_O20
  E : Outport
  wires:
  I/1 -> Kr*I/1, 2*Kr*I/1
  2*Kr*I/1 -> Sum/1
  Sum/1 -> p_H2/1
  Kr*I/1 -> Sum2/2
  n_airin/1 -> n_O2in/1
  Sum2/1 -> p_O2/1
  ln(p_O2)/1 -> 0.5ln(p_O2)/1
  0.5ln(p_O2)/1 -> Add/1
  ln(p_H2)/1 -> Add/2
  Add/1 -> E3/1
  n_H2in/1 -> Sum/2
  p_H2/1 -> Sum4/1
  p_O2/1 -> Sum3/2
  p_an0/1 -> Sum4/2
  p_cat0/1 -> Sum3/1
  Sum3/1 -> p_O2avg/1
  Sum4/1 -> p_H2avg/1
  n_O2in/1 -> Sum2/1
  Sum1/1 -> Product/1
  Product/1 -> E/1
  E-RH correlation/1 -> E-RH correlation1/1
  T/1 -> Product1/1, E0/1
  E-RH correlation1/1 -> Product/2
  E3/1 -> Product1/2
  Product1/1 -> Sum1/2
  E0/1 -> Sum1/1
  p_O2avg/1 -> ln(p_O2)/1
  p_H2avg/1 -> ln(p_H2)/1

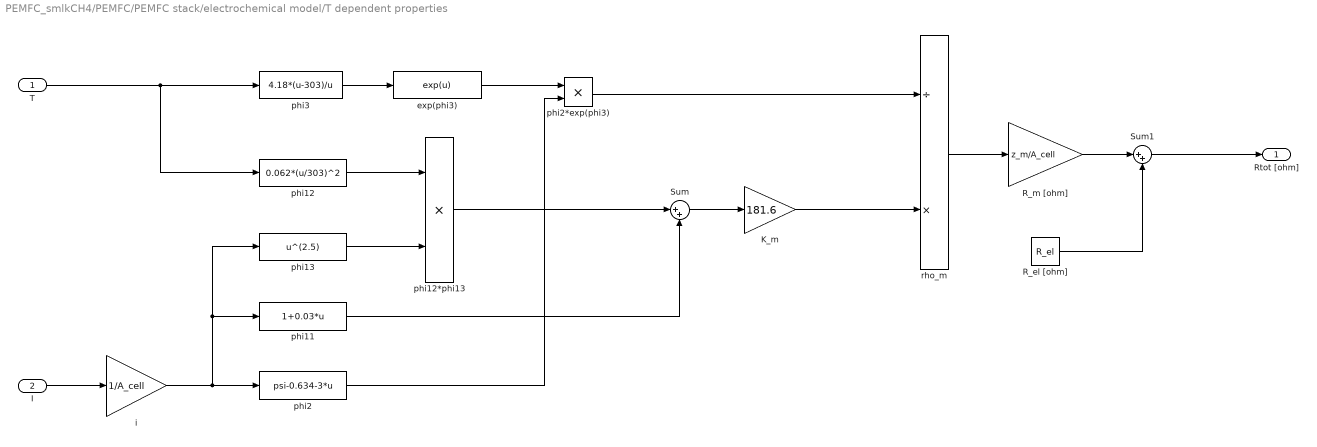
== system PEMFC_smlkCH4/PEMFC/PEMFC stack/electrochemical model/T dependent properties ==
  T : Inport
  I : Inport  Port=2
  K_m : Gain  Gain=181.6
  R_el [ohm] : Constant  Value=R_el
  R_m [ohm] : Gain  Gain=z_m/A_cell
  Sum : Sum  Inputs=|++
  Sum1 : Sum  Inputs=|++
  exp(phi3) : Fcn  Expr=exp(u)
  i : Gain  Gain=1/A_cell
  phi11 : Fcn  Expr=1+0.03*u
  phi12 : Fcn  Expr=0.062*(u/303)^2
  phi12*phi13 : Product
  phi13 : Fcn  Expr=u^(2.5)
  phi2 : Fcn  Expr=psi-0.634-3*u
  phi2*exp(phi3) : Product
  phi3 : Fcn  Expr=4.18*(u-303)/u
  rho_m : Product  Inputs=/*
  Rtot [ohm] : Outport
  wires:
  I/1 -> i/1
  i/1 -> phi13/1, phi11/1, phi2/1
  phi12/1 -> phi12*phi13/1
  phi13/1 -> phi12*phi13/2
  phi12*phi13/1 -> Sum/1
  phi11/1 -> Sum/2
  phi3/1 -> exp(phi3)/1
  exp(phi3)/1 -> phi2*exp(phi3)/1
  phi2/1 -> phi2*exp(phi3)/2
  Sum/1 -> K_m/1
  K_m/1 -> rho_m/2
  phi2*exp(phi3)/1 -> rho_m/1
  rho_m/1 -> R_m [ohm]/1
  R_m [ohm]/1 -> Sum1/1
  R_el [ohm]/1 -> Sum1/2
  Sum1/1 -> Rtot [ohm]/1
  T/1 -> phi3/1, phi12/1
